simulink model "SfSecurity"  (Simulink 6.0)
settings: Solver=ode5  SolverMode=SingleTasking  StartTime=0.0  StopTime=10000  FixedStep=.0001  RelTol=1e-3  AbsTol=1e-6
libraries: simulink x1
settings Model: CovMetricSettings=dcmtr  Creator=The MathWorks Inc.  LastModifiedBy=scaife  ExtModeTrigMode=oneshot  ExtModeArmWhenConnect=off  ExtModeAutoUpdateStatusClock=off
settings DataIOCC: LimitDataPoints=off  SaveOutput=off  SaveTime=off
settings OptimizationCC: BooleanDataType=off
settings DebuggingCC: CheckExecutionContextPreStartOutputMsg=on  CheckExecutionContextRuntimeOutputMsg=on  SolverPrmCheckMsg=none  IntegerOverflowMsg=none
settings HardwareCC: TargetUnknown=on
settings RTWCC: TemplateMakefile=grt_vc.tmf

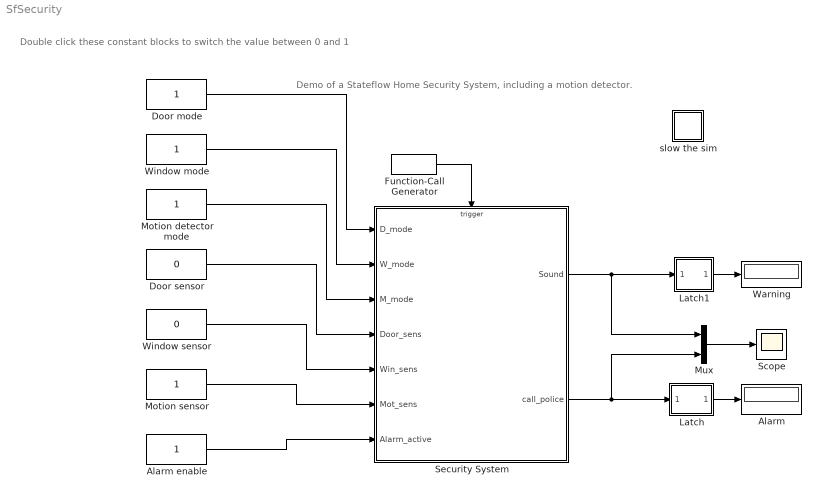
== system SfSecurity ==
  note: Demo of a Stateflow
      | Home Security System,
      | including a motion
      | detector.
  note: Double click these constant
      | blocks to switch the value
      | between 0 and 1
  Alarm : Display
  Alarm enable : Constant
      settings: OpenFcn=if strcmp(get_param(gcb,'value'),'1'), set_param(gcb,'value','0'); else set_param(gcb,'value','1'); end
  Door mode : Constant
      settings: OpenFcn=if strcmp(get_param(gcb,'value'),'1'), set_param(gcb,'value','0'); else set_param(gcb,'value','1'); end
  Door sensor : Constant  Value=0
      settings: OpenFcn=if strcmp(get_param(gcb,'value'),'1'), set_param(gcb,'value','0'); else set_param(gcb,'value','1'); end
  Function-Call Generator : simulink/Ports & Subsystems/Function-Call Generator  sample_time=.05  numberOfIterations=1
  Latch : Subsystem
      mask Display: disp('Hold')
  Latch1 : Subsystem
      mask Display: disp('Hold')
  Motion detector mode : Constant
      settings: OpenFcn=if strcmp(get_param(gcb,'value'),'1'), set_param(gcb,'value','0'); else set_param(gcb,'value','1'); end
  Motion sensor : Constant
      settings: OpenFcn=if strcmp(get_param(gcb,'value'),'1'), set_param(gcb,'value','0'); else set_param(gcb,'value','1'); end
  Mux : Mux  Inputs=2
  Scope : Scope
      settings: YMin=0  YMax=1  DataFormat=Structure
  Security System : Stateflow chart
  Warning : Display
  Window mode : Constant
      settings: OpenFcn=if strcmp(get_param(gcb,'value'),'1'), set_param(gcb,'value','0'); else set_param(gcb,'value','1'); end
  Window sensor : Constant  Value=0
      settings: OpenFcn=if strcmp(get_param(gcb,'value'),'1'), set_param(gcb,'value','0'); else set_param(gcb,'value','1'); end
  slow the sim : Subsystem
  wires:
  Latch/1(Trigger) -> Alarm/1
  Security System/1(Sound) -> Latch1/1(Reset), Mux/1
  Security System/2(call_police) -> Latch/1(Reset), Mux/2
  Door mode/1 -> Security System/1(D_mode)
  Window mode/1 -> Security System/2(W_mode)
  Motion detector mode/1 -> Security System/3(M_mode)
  Alarm enable/1 -> Security System/7(Alarm_active)
  Motion sensor/1 -> Security System/6(Mot_sens)
  Window sensor/1 -> Security System/5(Win_sens)
  Door sensor/1 -> Security System/4(Door_sens)
  Function-Call Generator/1 -> Security System/Trigger
  Mux/1 -> Scope/1
  Latch1/1(Trigger) -> Warning/1

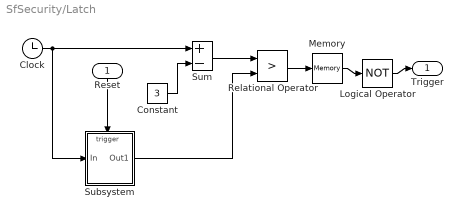
== system SfSecurity/Latch ==
  Reset : Inport  Orientation=down  Port=1  LatchInput=off
  Clock : Clock
      settings: Decimation=10
  Constant : Constant  Value=3
  Logical Operator : Logic  Operator=NOT  Inputs=1
  Memory : Memory  X0=1
  Relational Operator : RelationalOperator  Operator=>  InputSameDT=on
  Subsystem : Subsystem
  Sum : Sum  Inputs=+-  SaturateOnIntegerOverflow=on  InputSameDT=on
  Trigger : Outport  InitialOutput=0
  wires:
  Clock/1 -> Sum/1, Subsystem/1(In)
  Reset/1 -> Subsystem/Trigger
  Constant/1 -> Sum/2
  Sum/1 -> Relational Operator/1
  Subsystem/1(Out1) -> Relational Operator/2
  Relational Operator/1 -> Memory/1
  Memory/1 -> Logical Operator/1
  Logical Operator/1 -> Trigger/1

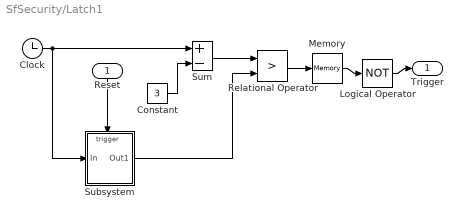
== system SfSecurity/Latch1 ==
  Reset : Inport  Orientation=down  Port=1  LatchInput=off
  Clock : Clock
      settings: Decimation=10
  Constant : Constant  Value=3
  Logical Operator : Logic  Operator=NOT  Inputs=1
  Memory : Memory  X0=1
  Relational Operator : RelationalOperator  Operator=>  InputSameDT=on
  Subsystem : Subsystem
  Sum : Sum  Inputs=+-  SaturateOnIntegerOverflow=on  InputSameDT=on
  Trigger : Outport  InitialOutput=0
  wires:
  Logical Operator/1 -> Trigger/1
  Memory/1 -> Logical Operator/1
  Relational Operator/1 -> Memory/1
  Subsystem/1(Out1) -> Relational Operator/2
  Sum/1 -> Relational Operator/1
  Constant/1 -> Sum/2
  Reset/1 -> Subsystem/Trigger
  Clock/1 -> Subsystem/1(In), Sum/1

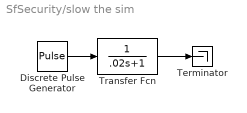
== system SfSecurity/slow the sim ==
  Discrete Pulse Generator : DiscretePulseGenerator  SampleTime=0.1
  Terminator : Terminator
  Transfer Fcn : TransferFcn  Denominator=[.02 1]
  wires:
  Discrete Pulse Generator/1 -> Transfer Fcn/1
  Transfer Fcn/1 -> Terminator/1

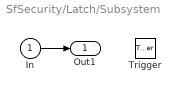
== system SfSecurity/Latch/Subsystem ==
  In : Inport  Port=1  LatchInput=off
  Trigger : TriggerPort  TriggerType=either
  Out1 : Outport  InitialOutput=-10
  wires:
  In/1 -> Out1/1

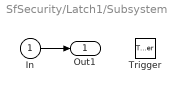
== system SfSecurity/Latch1/Subsystem ==
  In : Inport  Port=1  LatchInput=off
  Trigger : TriggerPort  TriggerType=either
  Out1 : Outport  InitialOutput=-10
  wires:
  In/1 -> Out1/1

== stateflow chart Security System ==
  state Motion [parallel]
    settings: description=This state models the modes of a motion detector sensor and implements logic to respond when that sensor is producing a signal.
    state Active
      state Idle
      state Debouncing
      Motion.Active.Idle -> Debouncing : [Mot_sens]
      Debouncing -> Debouncing : after(1/tSample,sl_call)
          | [ in(Alarm.On.Idle) ] /
          | send(Alert,Alarm);
      Debouncing -> Motion.Active.Idle : [!Mot_sens]
    state Disabled
      Motion.Disabled -> (junction 26) : [Mot_sens]
          | {send(Warn,Alarm);}
    (default) -> Motion.Active.Idle
      settings: description=On the first sample call the motion sensor mode is set to active, in the idle substate.
    Motion.Disabled -> Motion.Active.Idle : [M_mode==1]
    Motion.Active -> Motion.Disabled : [M_mode==0]
  state Win [parallel]
    settings: description=This state models the modes of a window sensor and implements logic to respond when that sensor is producing a signal.
    state Disabled
      Win.Disabled -> (junction 23) : [Win_sens]
          | {send(Warn,Alarm);}
    state Active
      Win.Active -> (junction 22) : [Win_sens && ...
          | in(Alarm.On.Idle)]
          | {send(Alert,Alarm);}
    Win.Active -> Win.Disabled : [W_mode==0]
    (default) -> Win.Active
      settings: description=On the first sample call the window mode is set to active.
    Win.Disabled -> Win.Active : [W_mode==1]
  state Alarm [parallel]
    state Off
    state On
      on  Warn: Sound;
      state Idle
      state Pending
        entry: Warn;
      Alarm.On.Idle -> Pending : Alert
      (default) -> Alarm.On.Idle
      Pending -> Alarm.On.Idle : after(2/tSample,sl_call)/
          | call_police;
    (default) -> On
      settings: description=On the first sample call the Alarm is set to active.
    Off -> On : [Alarm_active==1]
    On -> Off : [Alarm_active==0]
  state Door [parallel]
    settings: description=This state models the modes of a door sensor and implements logic to respond when that sensor is producing a signal.
    state Disabled
      Door.Disabled -> (junction 24) : [Door_sens]
          | {send(Warn,Alarm);}
    state Active
      Door.Active -> (junction 25) : [Door_sens && ...
          |  in(Alarm.On.Idle)]
          | {send(Alert,Alarm);}
    Door.Active -> Door.Disabled : [D_mode==0]
    (default) -> Door.Active
      settings: description=On the first sample call the door mode is set to active.
    Door.Disabled -> Door.Active : [D_mode==1]
  state When an Alert event is [group]
    broadcast to the Alarm
    state the pend state will
    be activated for a delay
    period.  If the alarm is not
    disabled during the delay
    period the police are
    contacted by the output
    event, call_police.
  state The Door and Win states read boolean status variables at each [group]
    update.  When the sensor variable is true a broadcast event is
    sent to the Alarm state.  If the the sensor is active, the Alert
    event is broadcast, otherwise the warn event is broadcast.
  state Input from the motion sensor can be sporadic [group]
    so a debounce state is used.  The debouncing
    state remains active while Mot_sens is true.
    After a delay period the Alert event is broadcast.
  data: D_mode input boolean; W_mode input boolean; M_mode input boolean; Door_sens input boolean; Win_sens input boolean; Mot_sens input boolean; Alarm_active input boolean; tSample constant double =0.5
  events: ACT local EITHER_EDGE_EVENT; DIS local EITHER_EDGE_EVENT; ACT local EITHER_EDGE_EVENT; DIS local EITHER_EDGE_EVENT; ACT local EITHER_EDGE_EVENT; DIS local EITHER_EDGE_EVENT; ACT local EITHER_EDGE_EVENT; DIS local EITHER_EDGE_EVENT; Sound output EITHER_EDGE_EVENT; call_police output EITHER_EDGE_EVENT; Warn local EITHER_EDGE_EVENT; Alert local EITHER_EDGE_EVENT; sl_call input FUNCTION_CALL_EVENT
